simulink model "SIM_nonlinear_LQR"  (R2016a)
settings: Solver=ode23t  SolverMode=SingleTasking  StartTime=0.0  StopTime=20  MaxStep=1e-4  RelTol=1e-3
undefined symbols (not defined in the file): K, Kr
settings Model: Creator=edzel  LastModifiedBy=edzel
settings DataIOCC: ReturnWorkspaceOutputs=on
settings DebuggingCC: UnconnectedInputMsg=none  UnconnectedOutputMsg=none  UnconnectedLineMsg=none  SFUnexpectedBacktrackingDiag=error  SFNoUnconditionalDefaultTransitionDiag=error
settings ModelReferenceCC: EnableRefExpFcnMdlSchedulingChecks=off
settings SFSimCC: SimUseLocalCustomCode=on
settings RTWCC: Description=Generic Real-Time Target  RTWUseLocalCustomCode=on
settings GRTTargetCC: TargetLangStandard=C99 (ISO)
settings ConfigComp: CovMetricSettings=dwe  CovSaveCumulativeToWorkspaceVar=off  CovSaveSingleToWorkspaceVar=off  CovExternalEMLEnable=on

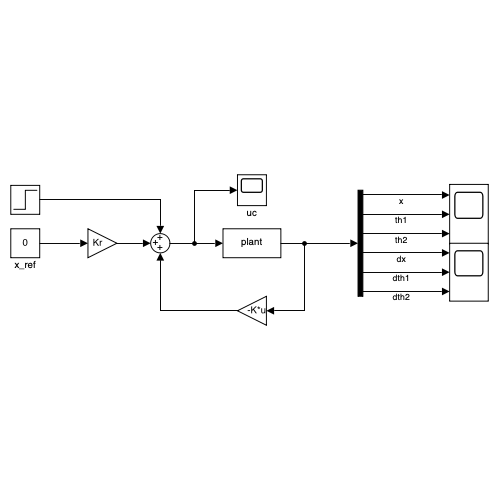
[thumbnail: Simulink's stored preview of the top-level diagram]
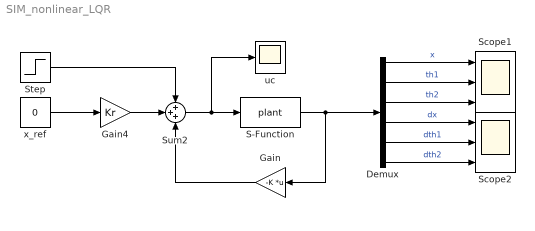
== system SIM_nonlinear_LQR ==
  Demux : Demux  Outputs=6
  Gain : Gain  Gain=-K  Multiplication=Matrix(K*u)
  Gain4 : Gain  Gain=Kr
  S-Function : S-Function  FunctionName=plant  Parameters=CoeF1, CoeF2, CoeF3, theta1_rad, theta2_rad  SFunctionDeploymentMode=off  EnableBusSupport=off
  Scope1 : Scope  NumInputPorts=3
  Scope2 : Scope  NumInputPorts=3
  Step : Step  Time=10  After=0.5  SampleTime=0
  Sum2 : Sum  Inputs=+++
  uc : Scope
  x_ref : Constant  Value=0
  wires:
  Demux/5 -> Scope2/2  "dth1"
  Demux/3 -> Scope1/3  "th2"
  Demux/1 -> Scope1/1  "x"
  Demux/2 -> Scope1/2  "th1"
  Demux/4 -> Scope2/1  "dx"
  Demux/6 -> Scope2/3  "dth2"
  S-Function/1 -> Demux/1, Gain/1
  Sum2/1 -> uc/1, S-Function/1
  x_ref/1 -> Gain4/1
  Step/1 -> Sum2/1
  Gain4/1 -> Sum2/2
  Gain/1 -> Sum2/3
